simulink model "ejercicioResorte"  (R2015a)
settings: Solver=ode45  StartTime=0.0  StopTime=100  RelTol=1e-3
undefined symbols (not defined in the file or in its folder): k1, k2, k3, m1, m2, m3
settings Model: Creator=Amanda  LastModifiedBy=Amanda

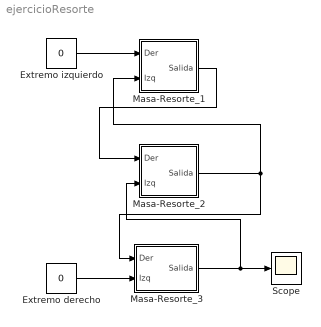
== system ejercicioResorte ==
  Extremo derecho : Constant  Value=0
  Extremo izquierdo : Constant  Value=0
  Masa-Resorte_1 : Subsystem
  Masa-Resorte_2 : Subsystem
  Masa-Resorte_3 : Subsystem
  Scope : Scope
  wires:
  Masa-Resorte_1/1(Salida) -> Masa-Resorte_2/1(Der)
  Masa-Resorte_2/1(Salida) -> Masa-Resorte_1/2(Izq), Masa-Resorte_3/1(Der)
  Masa-Resorte_3/1(Salida) -> Scope/1, Masa-Resorte_2/2(Izq)
  Extremo izquierdo/1 -> Masa-Resorte_1/1(Der)
  Extremo derecho/1 -> Masa-Resorte_3/2(Izq)

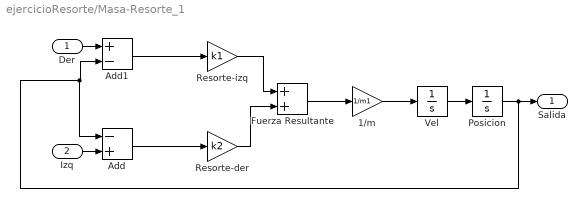
== system ejercicioResorte/Masa-Resorte_1 ==
  Der : Inport
  Izq : Inport  Port=2
  1/m : Gain  Gain=1/m1
  Add : Sum  Inputs=-+
  Add1 : Sum  Inputs=+-
  Fuerza Resultante : Sum
  Posicion : Integrator  InitialCondition=1
  Resorte-der : Gain  Gain=k2
  Resorte-izq : Gain  Gain=k1
  Vel : Integrator
  Salida : Outport
  wires:
  1/m/1 -> Vel/1
  Add/1 -> Resorte-der/1
  Add1/1 -> Resorte-izq/1
  Resorte-der/1 -> Fuerza Resultante/2
  Fuerza Resultante/1 -> 1/m/1
  Resorte-izq/1 -> Fuerza Resultante/1
  Vel/1 -> Posicion/1
  Posicion/1 -> Add/1, Add1/2, Salida/1
  Izq/1 -> Add/2
  Der/1 -> Add1/1

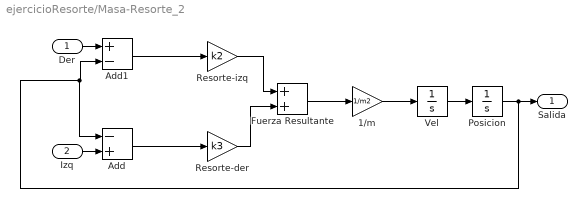
== system ejercicioResorte/Masa-Resorte_2 ==
  Der : Inport
  Izq : Inport  Port=2
  1/m : Gain  Gain=1/m2
  Add : Sum  Inputs=-+
  Add1 : Sum  Inputs=+-
  Fuerza Resultante : Sum
  Posicion : Integrator
  Resorte-der : Gain  Gain=k3
  Resorte-izq : Gain  Gain=k2
  Vel : Integrator
  Salida : Outport
  wires:
  1/m/1 -> Vel/1
  Add/1 -> Resorte-der/1
  Add1/1 -> Resorte-izq/1
  Resorte-der/1 -> Fuerza Resultante/2
  Fuerza Resultante/1 -> 1/m/1
  Resorte-izq/1 -> Fuerza Resultante/1
  Vel/1 -> Posicion/1
  Posicion/1 -> Add/1, Add1/2, Salida/1
  Izq/1 -> Add/2
  Der/1 -> Add1/1

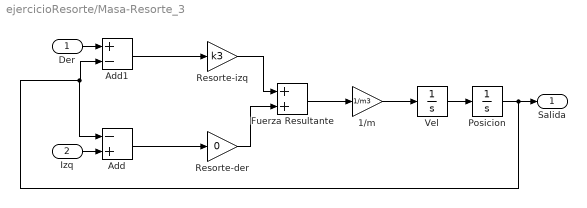
== system ejercicioResorte/Masa-Resorte_3 ==
  Der : Inport
  Izq : Inport  Port=2
  1/m : Gain  Gain=1/m3
  Add : Sum  Inputs=-+
  Add1 : Sum  Inputs=+-
  Fuerza Resultante : Sum
  Posicion : Integrator
  Resorte-der : Gain  Gain=0
  Resorte-izq : Gain  Gain=k3
  Vel : Integrator
  Salida : Outport
  wires:
  1/m/1 -> Vel/1
  Add/1 -> Resorte-der/1
  Add1/1 -> Resorte-izq/1
  Resorte-der/1 -> Fuerza Resultante/2
  Fuerza Resultante/1 -> 1/m/1
  Resorte-izq/1 -> Fuerza Resultante/1
  Vel/1 -> Posicion/1
  Posicion/1 -> Add/1, Add1/2, Salida/1
  Izq/1 -> Add/2
  Der/1 -> Add1/1
